simulink model "Dynamic_model"  (R2023a)
settings: Solver=VariableStepAuto  StartTime=0.0  StopTime=10.0  RelTol=1e-3
undefined symbols (not defined in the file): a, A_drag, b, B_drag, g, Ixx, Iyy, Izz, K, L, m, P0
settings Model: Creator=jonat  LastModifiedBy=jonat

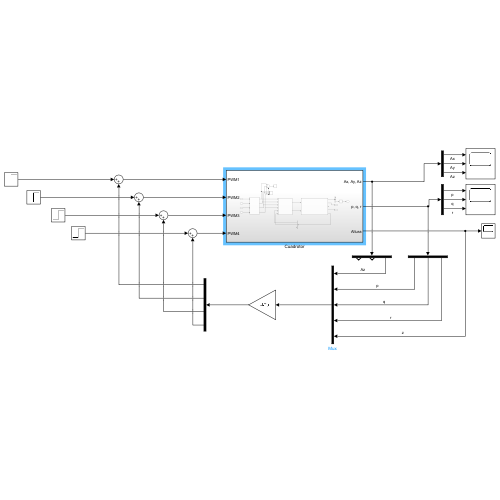
[thumbnail: Simulink's stored preview of the top-level diagram]
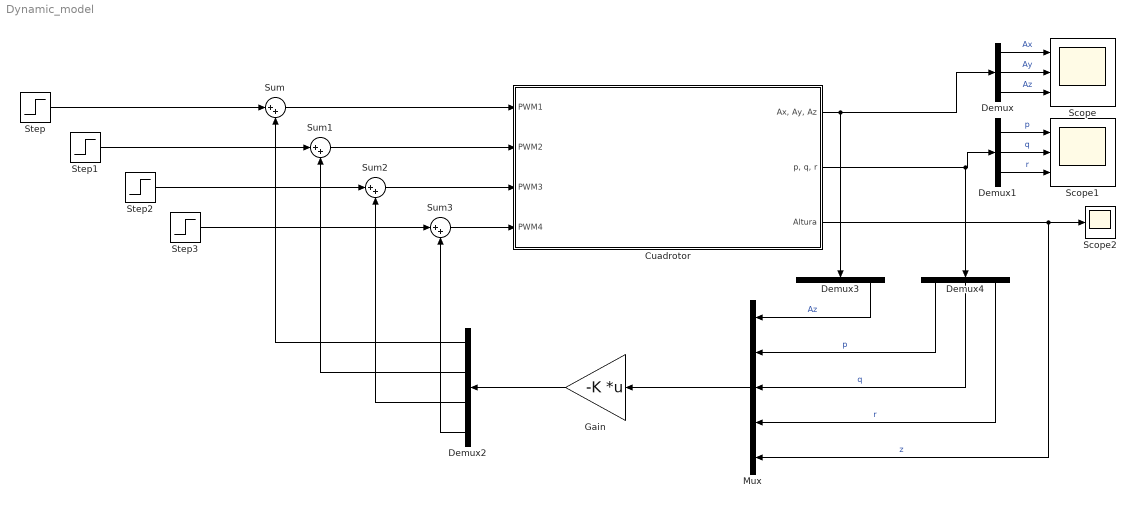
== system Dynamic_model ==
  Cuadrotor : Subsystem
  Demux{,1,3..4} (4 alike) : Demux  Outputs=3
  Demux2 : Demux
  Gain : Gain  Gain=-K  Multiplication=Matrix(K*u)
  Mux : Mux  Inputs=5
  Scope : Scope  NumInputPorts=3
  Scope1 : Scope  NumInputPorts=3
  Scope2 : Scope
  Step{,1..3} (4 alike) : Step  Time=0  After=P0  SampleTime=0
  Sum{,1..3} (4 alike) : Sum  Inputs=|++
  wires:
  Cuadrotor/3(Altura) -> Mux/5, Scope2/1  "z"
  Demux/1 -> Scope/1  "Ax"
  Demux/2 -> Scope/2  "Ay"
  Demux/3 -> Scope/3  "Az"
  Cuadrotor/1("Ax, Ay, Az") -> Demux3/1, Demux/1
  Cuadrotor/2("p, q, r") -> Demux1/1, Demux4/1
  Demux1/1 -> Scope1/1  "p"
  Demux1/2 -> Scope1/2  "q"
  Demux1/3 -> Scope1/3  "r"
  Step/1 -> Sum/1
  Sum/1 -> Cuadrotor/1(PWM1)
  Step1/1 -> Sum1/1
  Sum1/1 -> Cuadrotor/2(PWM2)
  Step2/1 -> Sum2/1
  Sum2/1 -> Cuadrotor/3(PWM3)
  Step3/1 -> Sum3/1
  Sum3/1 -> Cuadrotor/4(PWM4)
  Gain/1 -> Demux2/1
  Mux/1 -> Gain/1
  Demux2/1 -> Sum/2
  Demux2/2 -> Sum1/2
  Demux2/3 -> Sum2/2
  Demux2/4 -> Sum3/2
  Demux3/3 -> Mux/1  "Az"
  Demux4/1 -> Mux/2  "p"
  Demux4/2 -> Mux/3  "q"
  Demux4/3 -> Mux/4  "r"

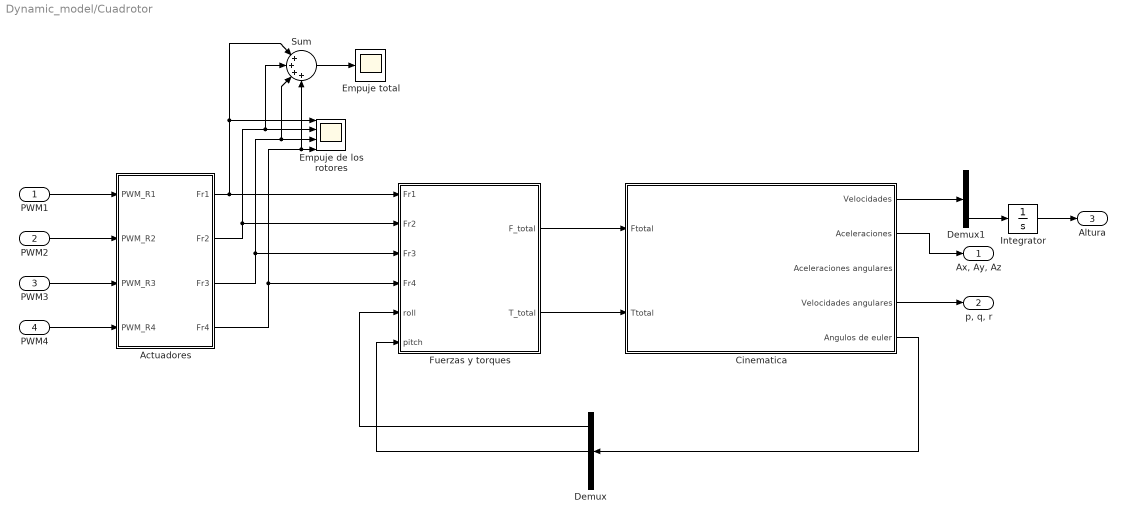
== system Dynamic_model/Cuadrotor ==
  PWM1 : Inport
  PWM2 : Inport  Port=2
  PWM3 : Inport  Port=3
  PWM4 : Inport  Port=4
  Actuadores : Subsystem
  Cinematica : Subsystem
  Demux : Demux  Outputs=3
  Demux1 : Demux  Outputs=3
  Empuje de los rotores : Scope  NumInputPorts=4
  Empuje total : Scope
  Fuerzas y torques : Subsystem
  Integrator : Integrator
  Sum : Sum  Inputs=|++++
  "Ax, Ay, Az" : Outport
  "p, q, r" : Outport  Port=2
  Altura : Outport  Port=3
  wires:
  PWM1/1 -> Actuadores/1(PWM_R1)
  PWM2/1 -> Actuadores/2(PWM_R2)
  PWM3/1 -> Actuadores/3(PWM_R3)
  PWM4/1 -> Actuadores/4(PWM_R4)
  Actuadores/1(Fr1) -> Sum/1, Empuje de los rotores/1, Fuerzas y torques/1(Fr1)
  Actuadores/2(Fr2) -> Fuerzas y torques/2(Fr2), Sum/2, Empuje de los rotores/2
  Actuadores/3(Fr3) -> Fuerzas y torques/3(Fr3), Sum/3, Empuje de los rotores/3
  Actuadores/4(Fr4) -> Fuerzas y torques/4(Fr4), Sum/4, Empuje de los rotores/4
  Sum/1 -> Empuje total/1
  Fuerzas y torques/1(F_total) -> Cinematica/1(Ftotal)
  Fuerzas y torques/2(T_total) -> Cinematica/2(Ttotal)
  Cinematica/5(Angulos de euler) -> Demux/1
  Demux/1 -> Fuerzas y torques/5(roll)
  Demux/2 -> Fuerzas y torques/6(pitch)
  Cinematica/4(Velocidades angulares) -> "p, q, r"/1
  Cinematica/1(Velocidades) -> Demux1/1
  Demux1/3 -> Integrator/1
  Integrator/1 -> Altura/1
  Cinematica/2(Aceleraciones) -> "Ax, Ay, Az"/1

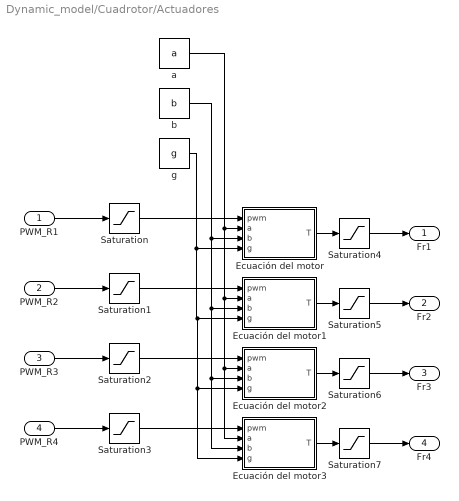
== system Dynamic_model/Cuadrotor/Actuadores ==
  PWM_R1 : Inport
  PWM_R2 : Inport  Port=2
  PWM_R3 : Inport  Port=3
  PWM_R4 : Inport  Port=4
  Ecuación del motor : MATLAB Function  TreatAsAtomicUnit=on
  Ecuación del motor1 : MATLAB Function  TreatAsAtomicUnit=on
  Ecuación del motor2 : MATLAB Function  TreatAsAtomicUnit=on
  Ecuación del motor3 : MATLAB Function  TreatAsAtomicUnit=on
  Saturation{,1..3} (4 alike) : Saturate  UpperLimit=0.002  LowerLimit=0.001
  Saturation{4..7} (4 alike) : Saturate  UpperLimit=10  LowerLimit=0
  a : Constant  Value=a
  b : Constant  Value=b
  g : Constant  Value=g
  Fr1 : Outport
  Fr2 : Outport  Port=2
  Fr3 : Outport  Port=3
  Fr4 : Outport  Port=4
  wires:
  PWM_R1/1 -> Saturation/1
  PWM_R2/1 -> Saturation1/1
  PWM_R3/1 -> Saturation2/1
  PWM_R4/1 -> Saturation3/1
  Saturation/1 -> Ecuación del motor/1(pwm)
  a/1 -> Ecuación del motor3/2(a), Ecuación del motor2/2(a), Ecuación del motor1/2(a), Ecuación del motor/2(a)
  b/1 -> Ecuación del motor/3(b), Ecuación del motor3/3(b), Ecuación del motor2/3(b), Ecuación del motor1/3(b)
  Ecuación del motor/1(T) -> Saturation4/1
  Ecuación del motor1/1(T) -> Saturation5/1
  Ecuación del motor2/1(T) -> Saturation6/1
  Ecuación del motor3/1(T) -> Saturation7/1
  Saturation1/1 -> Ecuación del motor1/1(pwm)
  Saturation2/1 -> Ecuación del motor2/1(pwm)
  Saturation3/1 -> Ecuación del motor3/1(pwm)
  Saturation7/1 -> Fr4/1
  Saturation6/1 -> Fr3/1
  Saturation5/1 -> Fr2/1
  Saturation4/1 -> Fr1/1
  g/1 -> Ecuación del motor3/4(g), Ecuación del motor2/4(g), Ecuación del motor1/4(g), Ecuación del motor/4(g)

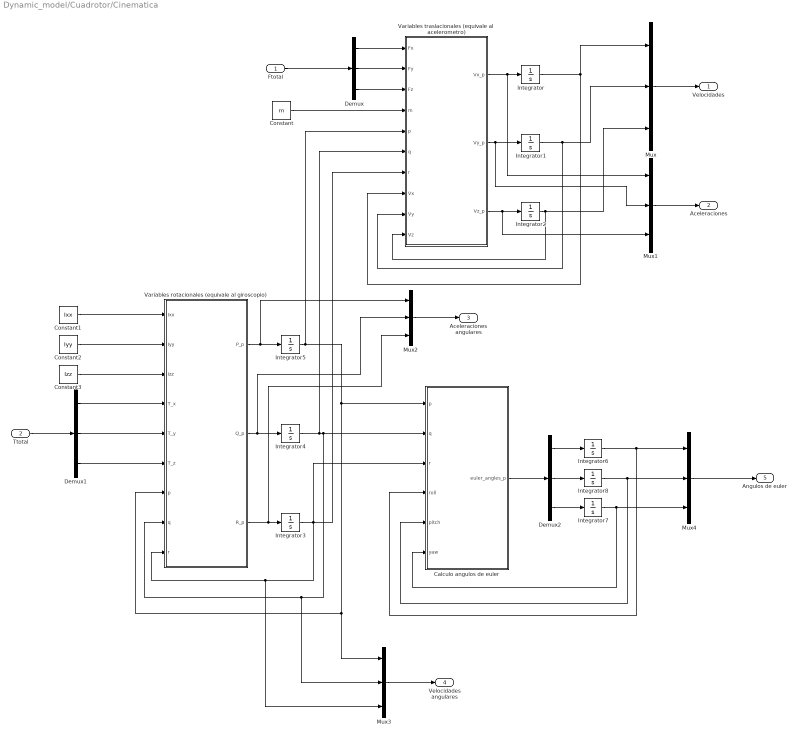
== system Dynamic_model/Cuadrotor/Cinematica ==
  Ftotal : Inport
  Ttotal : Inport  Port=2
  Calculo angulos de euler : MATLAB Function  TreatAsAtomicUnit=on
  Constant : Constant  Value=m
  Constant1 : Constant  Value=Ixx
  Constant2 : Constant  Value=Iyy
  Constant3 : Constant  Value=Izz
  Demux : Demux  Outputs=3
  Demux1 : Demux  Outputs=3
  Demux2 : Demux  Outputs=3
  Integrator{,1..8} (9 alike) : Integrator
  Mux{,1..4} (5 alike) : Mux  Inputs=3
  Variables rotacionales (equivale al giroscopio) : MATLAB Function  TreatAsAtomicUnit=on
  Variables traslacionales (equivale al acelerometro) : MATLAB Function  TreatAsAtomicUnit=on
  Velocidades : Outport
  Aceleraciones : Outport  Port=2
  Aceleraciones angulares : Outport  Port=3
  Velocidades angulares : Outport  Port=4
  Angulos de euler : Outport  Port=5
  wires:
  Ftotal/1 -> Demux/1
  Demux/1 -> Variables traslacionales (equivale al acelerometro)/1(Fx)
  Demux/2 -> Variables traslacionales (equivale al acelerometro)/2(Fy)
  Demux/3 -> Variables traslacionales (equivale al acelerometro)/3(Fz)
  Variables traslacionales (equivale al acelerometro)/1(Vx_p) -> Mux1/1, Integrator/1
  Variables traslacionales (equivale al acelerometro)/2(Vy_p) -> Mux1/2, Integrator1/1
  Variables traslacionales (equivale al acelerometro)/3(Vz_p) -> Mux1/3, Integrator2/1
  Integrator/1 -> Variables traslacionales (equivale al acelerometro)/8(Vx), Mux/1
  Integrator1/1 -> Variables traslacionales (equivale al acelerometro)/9(Vy), Mux/2
  Integrator2/1 -> Mux/3, Variables traslacionales (equivale al acelerometro)/10(Vz)
  Constant/1 -> Variables traslacionales (equivale al acelerometro)/4(m)
  Demux1/3 -> Variables rotacionales (equivale al giroscopio)/6(T_z)
  Demux1/2 -> Variables rotacionales (equivale al giroscopio)/5(T_y)
  Demux1/1 -> Variables rotacionales (equivale al giroscopio)/4(T_x)
  Ttotal/1 -> Demux1/1
  Constant1/1 -> Variables rotacionales (equivale al giroscopio)/1(Ixx)
  Constant2/1 -> Variables rotacionales (equivale al giroscopio)/2(Iyy)
  Constant3/1 -> Variables rotacionales (equivale al giroscopio)/3(Izz)
  Variables rotacionales (equivale al giroscopio)/1(P_p) -> Mux2/1, Integrator5/1
  Variables rotacionales (equivale al giroscopio)/2(Q_p) -> Mux2/2, Integrator4/1
  Variables rotacionales (equivale al giroscopio)/3(R_p) -> Mux2/3, Integrator3/1
  Integrator3/1 -> Variables traslacionales (equivale al acelerometro)/7(r), Mux3/3, Variables rotacionales (equivale al giroscopio)/9(r), Calculo angulos de euler/3(r)
  Integrator4/1 -> Variables traslacionales (equivale al acelerometro)/6(q), Calculo angulos de euler/2(q), Mux3/2, Variables rotacionales (equivale al giroscopio)/8(q)
  Integrator5/1 -> Variables traslacionales (equivale al acelerometro)/5(p), Calculo angulos de euler/1(p), Mux3/1, Variables rotacionales (equivale al giroscopio)/7(p)
  Calculo angulos de euler/1(euler_angles_p) -> Demux2/1
  Demux2/1 -> Integrator6/1
  Demux2/2 -> Integrator8/1
  Demux2/3 -> Integrator7/1
  Integrator7/1 -> Calculo angulos de euler/6(yaw), Mux4/3
  Integrator6/1 -> Calculo angulos de euler/4(roll), Mux4/1
  Mux/1 -> Velocidades/1
  Mux1/1 -> Aceleraciones/1
  Mux2/1 -> Aceleraciones angulares/1
  Mux3/1 -> Velocidades angulares/1
  Integrator8/1 -> Calculo angulos de euler/5(pitch), Mux4/2
  Mux4/1 -> Angulos de euler/1

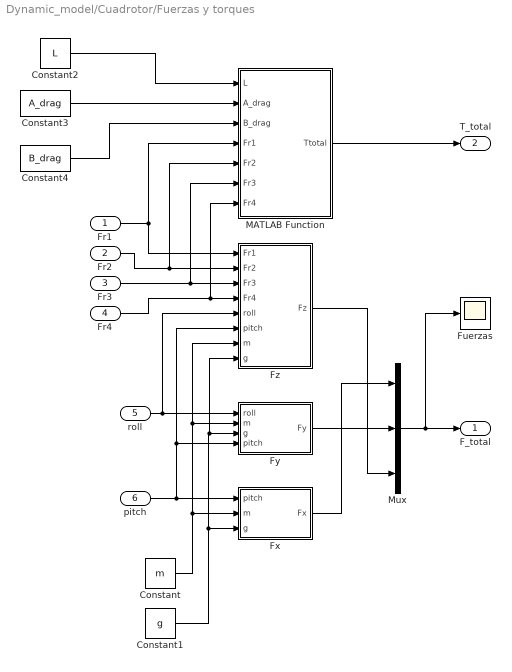
== system Dynamic_model/Cuadrotor/Fuerzas y torques ==
  Fr1 : Inport
  Fr2 : Inport  Port=2
  Fr3 : Inport  Port=3
  Fr4 : Inport  Port=4
  roll : Inport  Port=5
  pitch : Inport  Port=6
  Constant : Constant  Value=m
  Constant1 : Constant  Value=g
  Constant2 : Constant  Value=L
  Constant3 : Constant  Value=A_drag
  Constant4 : Constant  Value=B_drag
  Fuerzas : Scope
  Fx : MATLAB Function  TreatAsAtomicUnit=on
  Fy : MATLAB Function  TreatAsAtomicUnit=on
  Fz : MATLAB Function  TreatAsAtomicUnit=on
  MATLAB Function : MATLAB Function  TreatAsAtomicUnit=on
  Mux : Mux  Inputs=3
  F_total : Outport
  T_total : Outport  Port=2
  wires:
  pitch/1 -> Fy/4(pitch), Fz/6(pitch), Fx/1(pitch)
  Constant1/1 -> Fz/8(g), Fy/3(g), Fx/3(g)
  Constant/1 -> Fz/7(m), Fy/2(m), Fx/2(m)
  roll/1 -> Fy/1(roll), Fz/5(roll)
  Fr1/1 -> MATLAB Function/4(Fr1), Fz/1(Fr1)
  Fr2/1 -> MATLAB Function/5(Fr2), Fz/2(Fr2)
  Fr3/1 -> MATLAB Function/6(Fr3), Fz/3(Fr3)
  Fr4/1 -> MATLAB Function/7(Fr4), Fz/4(Fr4)
  Fx/1(Fx) -> Mux/1
  Fy/1(Fy) -> Mux/2
  Fz/1(Fz) -> Mux/3
  Mux/1 -> Fuerzas/1, F_total/1
  Constant3/1 -> MATLAB Function/2(A_drag)
  Constant2/1 -> MATLAB Function/1(L)
  Constant4/1 -> MATLAB Function/3(B_drag)
  MATLAB Function/1(Ttotal) -> T_total/1

== matlab function Dynamic_model/Cuadrotor/Cinematica/Variables traslacionales (equivale al acelerometro) ==
  data: Fx input; Vx_p output; Fy input; Fz input; m input; p input; q input; r input; Vx input; Vy input; Vz input; Vy_p output; Vz_p output
function [Vx_p, Vy_p, Vz_p] = fcn(Fx, Fy, Fz, m, p, q, r, Vx, Vy, Vz)

Vx_p = 1/m * (Fx - (q*Vz - r*Vy));
Vy_p = 1/m * (Fy - (r*Vx - p*Vz));
Vz_p = 1/m * (Fz - (p*Vz - q*Vx));

== matlab function Dynamic_model/Cuadrotor/Cinematica/Variables rotacionales (equivale al giroscopio) ==
  data: Ixx input; P_p output; Iyy input; Izz input; T_x input; T_y input; T_z input; p input; q input; r input; Q_p output; R_p output
function [P_p, Q_p, R_p] = fcn(Ixx, Iyy, Izz, T_x, T_y, T_z, p, q, r)

% Los torques se nombran como
% T_x = L
% T_y = M
% T_z = N
 
P_p = 1/Ixx * (T_x - (Izz - Iyy) * q * r);
Q_p = 1/Iyy * (T_y - (Ixx - Izz) * p * r);
R_p = 1/Izz * (T_z - (Iyy - Ixx) * p * q);

== matlab function Dynamic_model/Cuadrotor/Cinematica/Calculo angulos de euler ==
  data: p input; euler_angles_p output; q input; r input; roll input; pitch input; yaw input
function euler_angles_p = fcn(p, q, r, roll, pitch, yaw)

euler_angles_p = [1, sin(roll)*tan(pitch), cos(roll)*tan(pitch);
        0, cos(roll), -sin(roll)
        0, -sin(roll)/cos(pitch), cos(roll)/cos(pitch)] * [p; q; r];

== matlab function Dynamic_model/Cuadrotor/Actuadores/Ecuación del motor1 ==
  data: pwm input; T output; a input; b input; g input
function T = fcn(pwm, a, b, g)

T = (a*pwm + b)*g;

== matlab function Dynamic_model/Cuadrotor/Actuadores/Ecuación del motor ==
  data: pwm input; T output; a input; b input; g input
function T = fcn(pwm, a, b, g)

T = (a*pwm + b)*g;

% a va en kg

== matlab function Dynamic_model/Cuadrotor/Actuadores/Ecuación del motor2 ==
  data: pwm input; T output; a input; b input; g input
function T = fcn(pwm, a, b, g)

T = (a*pwm + b)*g;

== matlab function Dynamic_model/Cuadrotor/Actuadores/Ecuación del motor3 ==
  data: pwm input; T output; a input; b input; g input
function T = fcn(pwm, a, b, g)

T = (a*pwm + b)*g;

== matlab function Dynamic_model/Cuadrotor/Fuerzas y torques/Fx ==
  data: pitch input; m input; Fx output; g input
function Fx = fcn(pitch, m, g)

Fx = -m*g*sin(pitch);

== matlab function Dynamic_model/Cuadrotor/Fuerzas y torques/Fy ==
  data: roll input; m input; Fy output; g input; pitch input
function Fy = fcn(roll, m, g, pitch)

Fy = m*g*sin(roll)*cos(pitch);

== matlab function Dynamic_model/Cuadrotor/Fuerzas y torques/Fz ==
  data: Fr1 input; Fz output; Fr2 input; Fr3 input; Fr4 input; roll input; pitch input; m input; g input
function Fz = fcn(Fr1, Fr2, Fr3, Fr4, roll, pitch, m, g)

Fz = (Fr1 + Fr2 + Fr3 + Fr4) - (m*g*cos(roll)*cos(pitch));

== matlab function Dynamic_model/Cuadrotor/Fuerzas y torques/MATLAB Function ==
  data: L input; A_drag input; B_drag input; Ttotal output; Fr1 input; Fr2 input; Fr3 input; Fr4 input
function Ttotal  = fcn(L, A_drag, B_drag, Fr1, Fr2, Fr3, Fr4)

% Fr corresponde a las fuerzas de cada uno de los rotores

Tr1 = [L*Fr1; 0; 0];
Tr2 = [0; -L*Fr2; 0];
Tr3 = [-L*Fr3; 0; 0];
Tr4 = [0; L*Fr4; 0];

Qd1 = A_drag*(Fr1^(1.5)) + B_drag;
Qd2 = A_drag*(Fr2^(1.5)) + B_drag;
Qd3 = A_drag*(Fr3^(1.5)) + B_drag;
Qd4 = A_drag*(Fr4^(1.5)) + B_drag;

Td1 = [0; 0; Qd1];
Td2 = [0; 0; Qd2];
Td3 = [0; 0; Qd3];
Td4 = [0; 0; Qd4];

Ttotal = ((Tr1 - Td1 ) + (Tr3 - Td3)) - ((Tr2 - Td2) + (Tr4 - Td4));
